simulink model "Bipolar_SPWM"  (R2021a)
settings: Solver=ode23  StartTime=0.0  StopTime=.02*20  MaxStep=1e-4  RelTol=1e-3
model workspace (MAT data in the model file):
  Carrier_Frequency = 10050
  Carrier_Peak = 1
  Reference_Frequency = 50
  Reference_Peak = 1
libraries: spsIGBTDiodeLib x24, dsparch4 x6, spsRMSLib x6, spsThreePhaseVIMeasurementLib x6, spsDCVoltageSourceLib x4, spsTriangleGeneratorLib x4, spsVoltageMeasurementLib x4, spsAsynchronousMachineSIUnitsLib x2, spsGroundLib x2, spsThreePhaseSeriesRLCBranchLib x2, simulink x1, spspowerguiLib x1
settings Model: OrderedModelArguments=off  Creator=Ahmed Mohamed  LastModifiedBy=Ahmed Mohamed
settings SolverCC: AlgebraicLoopSolver=TrustRegion
settings DataIOCC: ReturnWorkspaceOutputs=off
settings DebuggingCC: SFMachineParentedDataDiag=warning

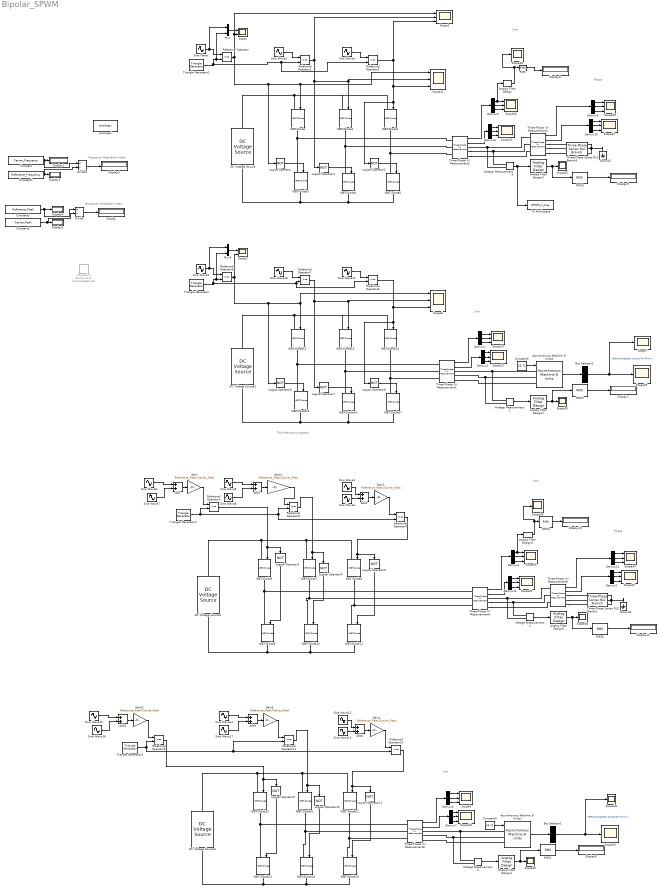
== system Bipolar_SPWM ==
  note: Third Harmonic Injection
  note: Amplitude Modulation Index
  note: Frequency Modulation Index
  note: Line
  note: Line
  note: Line
  note: Phase
  note: Line
  note: Phase
  Add{,1..5} (6 alike) : Sum
  Analog Filter Design : dsparch4/Analog Filter Design  method=Butterworth  filttype=Lowpass  N=8  Wlo=2*pi*500  Whi=80  Rp=2  Rs=40
  Analog Filter Design{1..3,5} (4 alike) : dsparch4/Analog Filter Design  method=Butterworth  filttype=Lowpass  N=8  Wlo=2*pi*1000  Whi=80  Rp=2  Rs=40
  Analog Filter Design4 : dsparch4/Analog Filter Design  method=Butterworth  filttype=Lowpass  N=8  Wlo=2*pi*500  Whi=80  Rp=2  Rs=40
  Asynchronous Machine SI Units1 : spsAsynchronousMachineSIUnitsLib/Asynchronous Machine SI Units  RotorType=Squirrel-cage  PresetModel="15:  5.4 HP (4KW)   400 V  50Hz 1430 RPM"  MechanicalLoad=Torque Tm  ShowDetailedParameters=on  ReferenceFrame=Rotor  Units=SI  MeasurementBus=off  NominalParameters=[4000 400 50]  VoltageRatio=1  Stator=[1.405 0.005839]  Rotor=[1.395 0.005839]  Cage1=[0.4155 0.002066]  Cage2=[0.4168 0.0003495]  Lm=0.1722  Mechanical=[0.0131 0.002985 2]  PolePairs=2  InitialConditions=[1 0 0 0 0 0 0 0]  SimulateSaturation=off  Saturation=[14.03593122, 27.81365428, 53.79336849, 72.68890987, 97.98006896, 148.6815601, 215.7428561, 302.9841135, 428.7778367 ; 230, 322, 414, 460, 506, 552, 598, 644, 690]  LoadFlowParameters=1492000  TsPowergui=0  TsBlock=-1  IterativeModel=Trapezoidal non iterative  IterativeDiscreteModel=Trapezoidal non iterative  Pmec=1.492e+006
  Asynchronous Machine SI Units2 : spsAsynchronousMachineSIUnitsLib/Asynchronous Machine SI Units  RotorType=Squirrel-cage  PresetModel="15:  5.4 HP (4KW)   400 V  50Hz 1430 RPM"  MechanicalLoad=Torque Tm  ShowDetailedParameters=on  ReferenceFrame=Rotor  Units=SI  MeasurementBus=off  NominalParameters=[4000 400 50]  VoltageRatio=1  Stator=[1.405 0.005839]  Rotor=[1.395 0.005839]  Cage1=[0.4155 0.002066]  Cage2=[0.4168 0.0003495]  Lm=0.1722  Mechanical=[0.0131 0.002985 2]  PolePairs=2  InitialConditions=[1 0 0 0 0 0 0 0]  SimulateSaturation=off  Saturation=[14.03593122, 27.81365428, 53.79336849, 72.68890987, 97.98006896, 148.6815601, 215.7428561, 302.9841135, 428.7778367 ; 230, 322, 414, 460, 506, 552, 598, 644, 690]  LoadFlowParameters=1492000  TsPowergui=0  TsBlock=-1  IterativeModel=Trapezoidal non iterative  IterativeDiscreteModel=Trapezoidal non iterative  Pmec=1.492e+006
  Bus Selector1 : BusSelector  OutputSignals=Mechanical.Electromagnetic torque Te (N*m)
  Bus Selector2 : BusSelector  OutputSignals=Mechanical.Electromagnetic torque Te (N*m)
  Constant : Constant  Value=Carrier_Frequency
  Constant1 : Constant  Value=Reference_Frequency
  Constant2 : Constant  Value=Carrier_Peak
  Constant3 : Constant  Value=Reference_Peak
  Constant4 : Constant  Value=26.71
  Constant5 : Constant  Value=26.71
  DC Voltage Source : spsDCVoltageSourceLib/DC Voltage Source  Amplitude=400*2*sqrt(2)/sqrt(3)  Measurements=None
  DC Voltage Source1 : spsDCVoltageSourceLib/DC Voltage Source  Amplitude=400*sqrt(2)/(sqrt(3)*1.15*.5)  Measurements=None
  DC Voltage Source2 : spsDCVoltageSourceLib/DC Voltage Source  Amplitude=400*2*sqrt(2)/sqrt(3)  Measurements=None
  DC Voltage Source3 : spsDCVoltageSourceLib/DC Voltage Source  Amplitude=400*sqrt(2)/(sqrt(3)*1.15*.5)  Measurements=None
  Demux{1..12} (12 alike) : Demux  Outputs=3
  Display{,1..11} (12 alike) : Display
  Divide : Product  Inputs=*/
  Divide1 : Product  Inputs=*/
  Gain{,1..5} (6 alike) : Gain  Gain=Reference_Peak/Carrier_Peak
  Ground1 : spsGroundLib/Ground  LConnTagsString=a
  Ground2 : spsGroundLib/Ground  LConnTagsString=a
  IGBT/Diode{,1..23} (24 alike) : spsIGBTDiodeLib/IGBT//Diode  Ron=1e-3  Rs=1e5  Cs=inf  Measurements=off
  Logical Operator{,1..11} (12 alike) : Logic  Operator=NOT  AllPortsSameDT=off  OutDataTypeStr=boolean
  Mux : Mux  Inputs=2
  Mux5 : Mux  Inputs=2
  RMS{,1..5} (6 alike) : spsRMSLib/RMS  TrueRMS=off  Freq=50  RMSInit=0  Ts=0
  Relational Operator{,1..11} (12 alike) : RelationalOperator  OutDataTypeStr=boolean  RndMeth=Simplest
  Repeating Sequence12 : simulink/Sources/Repeating Sequence  Commented=on  rep_seq_t=[0 .25/Carrier_Frequency .5/Carrier_Frequency .75/Carrier_Frequency 1/Carrier_Frequency]  rep_seq_y=[0 1 0 -1 0]
  Scope : Scope  NumInputPorts=2
  Scope{1,6,9,11,18,23..24,28..31,34..37} (15 alike) : Scope  NumInputPorts=3
  Scope{7,10,15..16,25..26,32..33,38..39} (10 alike) : Scope
  Scope2 : Scope  NumInputPorts=2
  Sine Wave : Sin  Amplitude=Reference_Peak  Frequency=2*Reference_Frequency*pi  SampleTime=0
  Sine Wave1 : Sin  Amplitude=Reference_Peak  Frequency=2*Reference_Frequency*pi  Phase=(2*pi)/3  SampleTime=0
  Sine Wave10 : Sin  Amplitude=Reference_Peak  Frequency=2*Reference_Frequency*pi  Phase=(2*pi)/3  SampleTime=0
  Sine Wave11 : Sin  Amplitude=Reference_Peak  Frequency=2*Reference_Frequency*pi  Phase=(4*pi)/3  SampleTime=0
  Sine Wave12 : Sin  Amplitude=1.15  Frequency=2*Reference_Frequency*pi  Phase=(4/3)*pi  SampleTime=0
  Sine Wave{4,7..8,13,16..17} (6 alike) : Sin  Amplitude=.19  Frequency=3*2*Reference_Frequency*pi  SampleTime=0
  Sine Wave14 : Sin  Amplitude=1.15  Frequency=2*Reference_Frequency*pi  Phase=(2/3)*pi  SampleTime=0
  Sine Wave15 : Sin  Amplitude=1.15  Frequency=2*Reference_Frequency*pi  SampleTime=0
  Sine Wave2 : Sin  Amplitude=Reference_Peak  Frequency=2*Reference_Frequency*pi  Phase=(4*pi)/3  SampleTime=0
  Sine Wave3 : Sin  Amplitude=1.15  Frequency=2*Reference_Frequency*pi  Phase=(4/3)*pi  SampleTime=0
  Sine Wave5 : Sin  Amplitude=1.15  Frequency=2*Reference_Frequency*pi  Phase=(2/3)*pi  SampleTime=0
  Sine Wave6 : Sin  Amplitude=1.15  Frequency=2*Reference_Frequency*pi  SampleTime=0
  Sine Wave9 : Sin  Amplitude=Reference_Peak  Frequency=2*Reference_Frequency*pi  SampleTime=0
  Three-Phase Series RLC Branch1 : spsThreePhaseSeriesRLCBranchLib/Three-Phase Series RLC Branch  LConnTagsString=A|B|C  RConnTagsString=A|B|C  BranchType=RL  Resistance=7.5*sqrt(2)  Inductance=7.5*sqrt(2)/314  Capacitance=1e-6  Measurements=None
  Three-Phase Series RLC Branch3 : spsThreePhaseSeriesRLCBranchLib/Three-Phase Series RLC Branch  LConnTagsString=A|B|C  RConnTagsString=A|B|C  BranchType=RL  Resistance=7.5*sqrt(2)  Inductance=7.5*sqrt(2)/314  Capacitance=1e-6  Measurements=None
  Three-Phase V-I Measurement{1..2,4,8} (4 alike) : spsThreePhaseVIMeasurementLib/Three-Phase V-I Measurement  VoltageMeasurement=phase-to-phase  SetLabelV=off  LabelV=Vabc  Vpu=off  VpuLL=off  CurrentMeasurement=yes  SetLabelI=off  LabelI=Iabc  Ipu=off  Pbase=100e6  Vbase=500e3  OutputType=Complex  PhasorSimulation=off  PSBequivalent=0
  Three-Phase V-I Measurement3 : spsThreePhaseVIMeasurementLib/Three-Phase V-I Measurement  VoltageMeasurement=phase-to-ground  SetLabelV=off  LabelV=Vabc  Vpu=off  VpuLL=off  CurrentMeasurement=yes  SetLabelI=off  LabelI=Iabc  Ipu=off  Pbase=100e6  Vbase=500e3  OutputType=Complex  PhasorSimulation=off  PSBequivalent=0
  Three-Phase V-I Measurement5 : spsThreePhaseVIMeasurementLib/Three-Phase V-I Measurement  VoltageMeasurement=phase-to-ground  SetLabelV=off  LabelV=Vabc  Vpu=off  VpuLL=off  CurrentMeasurement=yes  SetLabelI=off  LabelI=Iabc  Ipu=off  Pbase=100e6  Vbase=500e3  OutputType=Complex  PhasorSimulation=off  PSBequivalent=0
  To Workspace : ToWorkspace  VariableName=SPWM_V_Line  SaveFormat=Structure With Time  SampleTime=-1
  Triangle Generator{,1..3} (4 alike) : spsTriangleGeneratorLib/Triangle Generator  Freq=Carrier_Frequency  Phase=90  Ts=0
  Voltage Measurement{1..4} (4 alike) : spsVoltageMeasurementLib/Voltage Measurement  PhasorSimulation=off  OutputType=Complex  PSBequivalent=0
  powergui : spspowerguiLib/powergui  Priority=1  SimulationMode=Discrete  SampleTime=1e-6  frequency=60  Iterations=50  frequencyindice=0  Pbase=100e6  ErrMax=1e-4  UnitsV=kV  UnitsW=MW  buscounter=0  FunctionMessages=off  echomessages=off  EnableUseOfTLC=off  CurrentSourceSwitches=off  DisableSnubberDevices=off  DisableRonSwitches=off  DisableVfSwitches=off  DisplayEquations=off  AutomaticDiscreteSolvers=off  SolverType=Tustin/Backward Euler (TBE)  Interpol=off  ExternalGateDelay=off  methode=off  Ts=100  x0status=blocks  SPID=on  SwTol=0  HookPort=off  NonlinearTolerance=1e-4  nMaxIteration=100  ContinueOnMaxIteration=off  RestoreLinks=warning  ResistiveCurrentMeasurement=off  Frange=[0:2:500]  Ylog=off  Xlog=on  ShowGrid=off  save=off  variable=ZData  structure=Third_harmonic_injection_Bipolar_SPWM_Vline_out  ZoomFFT=off  StartTime=.16  cycles=1  DisplayStyle=1  fundamental=50  FreqAxis=off  MaxFrequency=1000  frequencyindicesteady=1  RmsSteady=1  display=off
  wires:
  Sine Wave/1 -> Mux/1, Relational Operator/1
  Mux/1 -> Scope/1
  Relational Operator/1 -> Logical Operator/1, Scope11/1, IGBT/Diode/1, Scope1/1, Scope/2
  Sine Wave1/1 -> Relational Operator1/1
  Logical Operator/1 -> IGBT/Diode3/1
  Logical Operator1/1 -> IGBT/Diode4/1
  Logical Operator2/1 -> IGBT/Diode5/1
  Sine Wave2/1 -> Relational Operator2/1
  Triangle Generator1/1 -> Relational Operator2/2, Relational Operator1/2, Mux/2, Relational Operator/2
  Relational Operator1/1 -> IGBT/Diode1/1, Scope11/2, Logical Operator1/1, Scope1/2
  Constant1/1 -> Divide1/2, Display2/1
  Constant/1 -> Divide1/1, Display1/1
  Divide/1 -> Display/1
  Constant3/1 -> Divide/1, Display4/1
  Constant2/1 -> Divide/2, Display3/1
  Divide1/1 -> Display5/1
  Relational Operator4/1 -> IGBT/Diode8/1, Logical Operator5/1
  Logical Operator5/1 -> IGBT/Diode11/1
  Logical Operator4/1 -> IGBT/Diode10/1
  Logical Operator3/1 -> IGBT/Diode9/1
  Relational Operator3/1 -> IGBT/Diode6/1, Logical Operator3/1
  Sine Wave6/1 -> Add/1
  Sine Wave7/1 -> Add/2
  Add/1 -> Gain/1
  Gain/1 -> Relational Operator3/1
  Gain1/1 -> Relational Operator4/1
  Add1/1 -> Gain1/1
  Sine Wave4/1 -> Add1/2
  Sine Wave3/1 -> Add1/1
  Triangle Generator2/1 -> Relational Operator5/2, Relational Operator4/2, Relational Operator3/2
  Gain2/1 -> Relational Operator5/1
  Add2/1 -> Gain2/1
  Sine Wave8/1 -> Add2/2
  Sine Wave5/1 -> Add2/1
  Relational Operator5/1 -> Logical Operator4/1, IGBT/Diode7/1
  Relational Operator8/1 -> IGBT/Diode14/1, Logical Operator8/1, Scope6/3
  Relational Operator7/1 -> Logical Operator7/1, Scope6/2, IGBT/Diode13/1
  Triangle Generator/1 -> Relational Operator8/2, Relational Operator7/2, Relational Operator6/2, Mux5/2
  Sine Wave11/1 -> Relational Operator8/1
  Logical Operator8/1 -> IGBT/Diode17/1
  Logical Operator7/1 -> IGBT/Diode16/1
  Logical Operator6/1 -> IGBT/Diode15/1
  Sine Wave10/1 -> Relational Operator7/1
  Relational Operator6/1 -> Scope2/2, IGBT/Diode12/1, Scope6/1, Logical Operator6/1
  Mux5/1 -> Scope2/1
  Sine Wave9/1 -> Relational Operator6/1, Mux5/1
  Relational Operator11/1 -> IGBT/Diode21/1, Logical Operator10/1
  Sine Wave14/1 -> Add5/1
  Sine Wave17/1 -> Add5/2
  Add5/1 -> Gain5/1
  Gain5/1 -> Relational Operator11/1
  Triangle Generator3/1 -> Relational Operator9/2, Relational Operator11/2, Relational Operator10/2
  Sine Wave12/1 -> Add4/1
  Sine Wave13/1 -> Add4/2
  Add4/1 -> Gain4/1
  Gain4/1 -> Relational Operator10/1
  Gain3/1 -> Relational Operator9/1
  Add3/1 -> Gain3/1
  Sine Wave16/1 -> Add3/2
  Sine Wave15/1 -> Add3/1
  Relational Operator9/1 -> Logical Operator9/1, IGBT/Diode20/1
  Logical Operator9/1 -> IGBT/Diode23/1
  Logical Operator10/1 -> IGBT/Diode18/1
  Logical Operator11/1 -> IGBT/Diode19/1
  Relational Operator10/1 -> Logical Operator11/1, IGBT/Diode22/1
  Voltage Measurement2/1 -> Analog Filter Design1/1
  Demux7/2 -> Scope18/2
  Demux6/3 -> Scope9/3
  Demux6/1 -> Scope9/1
  Demux6/2 -> Scope9/2
  Constant4/1 -> Asynchronous Machine SI Units2/1
  Asynchronous Machine SI Units2/1 -> Bus Selector1/1
  Three-Phase V-I Measurement8/1 -> Demux6/1
  Demux7/3 -> Scope18/3
  Demux7/1 -> Scope18/1
  Three-Phase V-I Measurement8/2 -> Demux7/1
  RMS1/1 -> Display6/1
  Analog Filter Design1/1 -> Scope15/1, RMS1/1
  Bus Selector1/1 -> Scope16/1, Scope10/1  "<Electromagnetic torque Te (N*m)>"
  Voltage Measurement1/1 -> Analog Filter Design2/1
  Demux2/2 -> Scope23/2
  Demux1/3 -> Scope24/3
  Demux1/1 -> Scope24/1
  Demux1/2 -> Scope24/2
  Constant5/1 -> Asynchronous Machine SI Units1/1
  Asynchronous Machine SI Units1/1 -> Bus Selector2/1
  Three-Phase V-I Measurement1/1 -> Demux1/1
  Demux2/3 -> Scope23/3
  Demux2/1 -> Scope23/1
  Three-Phase V-I Measurement1/2 -> Demux2/1
  RMS2/1 -> Display7/1
  Analog Filter Design2/1 -> Scope26/1, RMS2/1
  Bus Selector2/1 -> Scope7/1, Scope25/1  "<Electromagnetic torque Te (N*m)>"
  Analog Filter Design/1 -> Scope33/1, RMS/1
  Demux8/3 -> Scope29/3
  Demux9/1 -> Scope28/1
  RMS/1 -> Display8/1
  Three-Phase V-I Measurement2/1 -> Demux5/1
  Demux8/2 -> Scope29/2
  Three-Phase V-I Measurement2/2 -> Demux8/1
  Demux9/2 -> Scope28/2
  Demux8/1 -> Scope29/1
  Demux10/2 -> Scope31/2
  Voltage Measurement3/1 -> To Workspace/1, Analog Filter Design3/1
  RMS3/1 -> Display9/1
  Three-Phase V-I Measurement3/1 -> Demux9/1
  Analog Filter Design3/1 -> RMS3/1, Scope32/1
  Demux5/2 -> Scope30/2
  Three-Phase V-I Measurement3/2 -> Demux10/1
  Demux9/3 -> Scope28/3
  Demux10/3 -> Scope31/3
  Demux5/1 -> Scope30/1, Analog Filter Design/1
  Demux5/3 -> Scope30/3
  Demux10/1 -> Scope31/1
  Analog Filter Design4/1 -> Scope39/1, RMS4/1
  Demux11/3 -> Scope35/3
  Demux12/1 -> Scope34/1
  RMS4/1 -> Display10/1
  Three-Phase V-I Measurement4/1 -> Demux4/1
  Demux11/2 -> Scope35/2
  Three-Phase V-I Measurement4/2 -> Demux11/1
  Demux12/2 -> Scope34/2
  Demux11/1 -> Scope35/1
  Demux3/2 -> Scope37/2
  Voltage Measurement4/1 -> Analog Filter Design5/1
  RMS5/1 -> Display11/1
  Three-Phase V-I Measurement5/1 -> Demux12/1
  Analog Filter Design5/1 -> RMS5/1, Scope38/1
  Demux4/2 -> Scope36/2
  Three-Phase V-I Measurement5/2 -> Demux3/1
  Demux12/3 -> Scope34/3
  Demux3/3 -> Scope37/3
  Demux4/1 -> Scope36/1, Analog Filter Design4/1
  Demux4/3 -> Scope36/3
  Demux3/1 -> Scope37/1
  Relational Operator2/1 -> Scope11/3, Logical Operator2/1, IGBT/Diode2/1, Scope1/3
  connections:
  IGBT/Diode/RConn1 -- Three-Phase V-I Measurement2/LConn1 -- IGBT/Diode3/LConn1
  DC Voltage Source/RConn1 -- IGBT/Diode2/LConn1 -- IGBT/Diode1/LConn1 -- IGBT/Diode/LConn1
  IGBT/Diode5/RConn1 -- DC Voltage Source/LConn1 -- IGBT/Diode3/RConn1 -- IGBT/Diode4/RConn1
  IGBT/Diode6/RConn1 -- Three-Phase V-I Measurement4/LConn1 -- IGBT/Diode9/LConn1
  IGBT/Diode7/RConn1 -- Three-Phase V-I Measurement4/LConn2 -- IGBT/Diode10/LConn1
  IGBT/Diode8/RConn1 -- IGBT/Diode11/LConn1 -- Three-Phase V-I Measurement4/LConn3
  IGBT/Diode8/LConn1 -- IGBT/Diode7/LConn1 -- IGBT/Diode6/LConn1 -- DC Voltage Source1/RConn1
  IGBT/Diode10/RConn1 -- DC Voltage Source1/LConn1 -- IGBT/Diode9/RConn1 -- IGBT/Diode11/RConn1
  IGBT/Diode1/RConn1 -- Three-Phase V-I Measurement2/LConn2 -- IGBT/Diode4/LConn1
  IGBT/Diode2/RConn1 -- Three-Phase V-I Measurement2/LConn3 -- IGBT/Diode5/LConn1
  DC Voltage Source2/RConn1 -- IGBT/Diode12/LConn1 -- IGBT/Diode13/LConn1 -- IGBT/Diode14/LConn1
  IGBT/Diode17/RConn1 -- IGBT/Diode15/RConn1 -- DC Voltage Source2/LConn1 -- IGBT/Diode16/RConn1
  IGBT/Diode13/RConn1 -- Three-Phase V-I Measurement1/LConn2 -- IGBT/Diode16/LConn1
  IGBT/Diode14/RConn1 -- Three-Phase V-I Measurement1/LConn3 -- IGBT/Diode17/LConn1
  IGBT/Diode12/RConn1 -- Three-Phase V-I Measurement1/LConn1 -- IGBT/Diode15/LConn1
  IGBT/Diode22/LConn1 -- DC Voltage Source3/RConn1 -- IGBT/Diode20/LConn1 -- IGBT/Diode21/LConn1
  IGBT/Diode18/RConn1 -- IGBT/Diode19/RConn1 -- IGBT/Diode23/RConn1 -- DC Voltage Source3/LConn1
  IGBT/Diode22/RConn1 -- Three-Phase V-I Measurement8/LConn3 -- IGBT/Diode19/LConn1
  IGBT/Diode21/RConn1 -- Three-Phase V-I Measurement8/LConn2 -- IGBT/Diode18/LConn1
  IGBT/Diode20/RConn1 -- Three-Phase V-I Measurement8/LConn1 -- IGBT/Diode23/LConn1
  Asynchronous Machine SI Units2/LConn2 -- Voltage Measurement2/LConn2 -- Three-Phase V-I Measurement8/RConn2
  Asynchronous Machine SI Units2/LConn1 -- Voltage Measurement2/LConn1 -- Three-Phase V-I Measurement8/RConn1
  Asynchronous Machine SI Units2/LConn3 -- Three-Phase V-I Measurement8/RConn3
  Asynchronous Machine SI Units1/LConn2 -- Voltage Measurement1/LConn2 -- Three-Phase V-I Measurement1/RConn2
  Asynchronous Machine SI Units1/LConn1 -- Voltage Measurement1/LConn1 -- Three-Phase V-I Measurement1/RConn1
  Asynchronous Machine SI Units1/LConn3 -- Three-Phase V-I Measurement1/RConn3
  Three-Phase Series RLC Branch3/RConn2 -- Three-Phase Series RLC Branch3/RConn3 -- Three-Phase Series RLC Branch3/RConn1 -- Ground1/LConn1
  Three-Phase V-I Measurement2/RConn2 -- Voltage Measurement3/LConn1 -- Three-Phase V-I Measurement3/LConn2
  Three-Phase V-I Measurement3/LConn1 -- Voltage Measurement3/LConn2 -- Three-Phase V-I Measurement2/RConn1
  Three-Phase V-I Measurement3/RConn2 -- Three-Phase Series RLC Branch3/LConn2
  Three-Phase V-I Measurement3/RConn3 -- Three-Phase Series RLC Branch3/LConn3
  Three-Phase V-I Measurement2/RConn3 -- Three-Phase V-I Measurement3/LConn3
  Three-Phase V-I Measurement3/RConn1 -- Three-Phase Series RLC Branch3/LConn1
  Three-Phase Series RLC Branch1/RConn2 -- Three-Phase Series RLC Branch1/RConn3 -- Three-Phase Series RLC Branch1/RConn1 -- Ground2/LConn1
  Three-Phase V-I Measurement4/RConn2 -- Voltage Measurement4/LConn1 -- Three-Phase V-I Measurement5/LConn2
  Three-Phase V-I Measurement5/LConn1 -- Voltage Measurement4/LConn2 -- Three-Phase V-I Measurement4/RConn1
  Three-Phase V-I Measurement5/RConn2 -- Three-Phase Series RLC Branch1/LConn2
  Three-Phase V-I Measurement5/RConn3 -- Three-Phase Series RLC Branch1/LConn3
  Three-Phase V-I Measurement4/RConn3 -- Three-Phase V-I Measurement5/LConn3
  Three-Phase V-I Measurement5/RConn1 -- Three-Phase Series RLC Branch1/LConn1
